simulink model "icrf_unit"  (R2023b)
settings: Solver=VariableStepAuto  StartTime=0.0  StopTime=10.0  RelTol=1e-3
libraries: matrix_library x2, vrlib x2
settings Model: Creator=miqui  LastModifiedBy=miqui

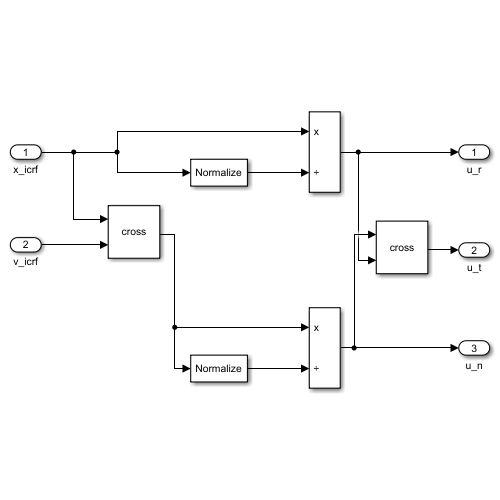
[thumbnail: Simulink's stored preview of the top-level diagram]
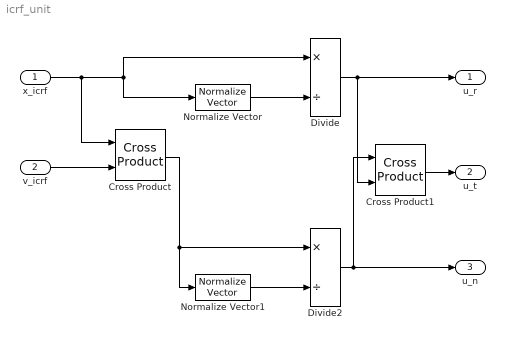
== system icrf_unit ==
  x_icrf : Inport
  v_icrf : Inport  Port=2
  Cross Product : matrix_library/Cross Product
  Cross Product1 : matrix_library/Cross Product
  Divide : Product  Inputs=*/
  Divide2 : Product  Inputs=*/
  Normalize Vector : vrlib/Utilities/Normalize Vector  maxzero=0
  Normalize Vector1 : vrlib/Utilities/Normalize Vector  maxzero=0
  u_r : Outport
  u_t : Outport  Port=2
  u_n : Outport  Port=3
  wires:
  Cross Product/1 -> Normalize Vector1/1, Divide2/1
  Normalize Vector1/1 -> Divide2/2
  Cross Product1/1 -> u_t/1
  Divide/1 -> Cross Product1/2, u_r/1
  v_icrf/1 -> Cross Product/2
  x_icrf/1 -> Cross Product/1, Normalize Vector/1, Divide/1
  Normalize Vector/1 -> Divide/2
  Divide2/1 -> Cross Product1/1, u_n/1
